simulink model "CITRIS_original"  (Simulink 7.4)
settings: Solver=FixedStepDiscrete  StartTime=0.0  StopTime=20  FixedStep=1  MaxStep=1  RelTol=1e-3
values from neighbouring files (symbols this model uses):
  mdot = [mdot controlInputHistory{i}(1,:)']    [CITRISBLOMSimulation.m]
  mdotmax = 740    [CITRISBLOMSimulation.m]
  mdotmin = 220    [CITRISBLOMSimulation.m]
  model =     [model.mat]
  vlv = [vlv controlInputHistory{i}(2,:)']    [CITRISBLOMSimulation.m]
undefined symbols (not defined in the file or in its folder): i, mdotTk, mdotvlv, mdotvlvk, Tk, TmaxSlack, TmaxV, TminSlack, TminV, wk, wk_1, wk_2
libraries: MPCMdlLib x19
settings Model: Creator=vichik  LastModifiedBy=Kyle
settings OptimizationCC: InitFltsAndDblsToZero=on

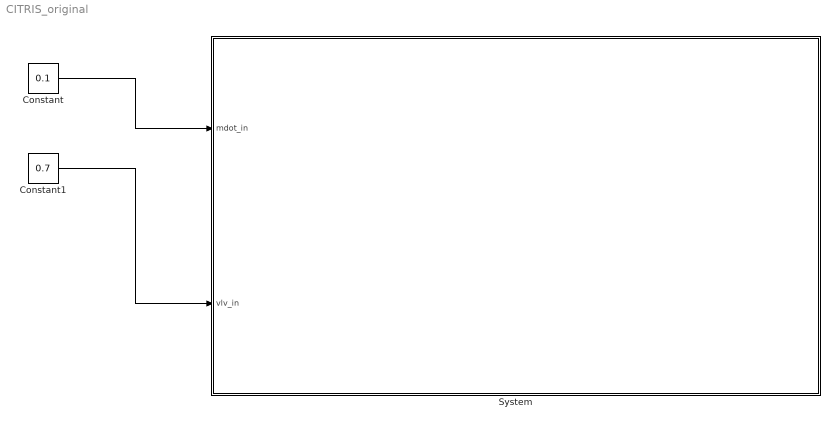
== system CITRIS_original ==
  Constant : Constant  Value=0.1
  Constant1 : Constant  Value=0.7
  System : Subsystem
  wires:
  Constant/1 -> System/1(mdot_in)
  Constant1/1 -> System/2(vlv_in)

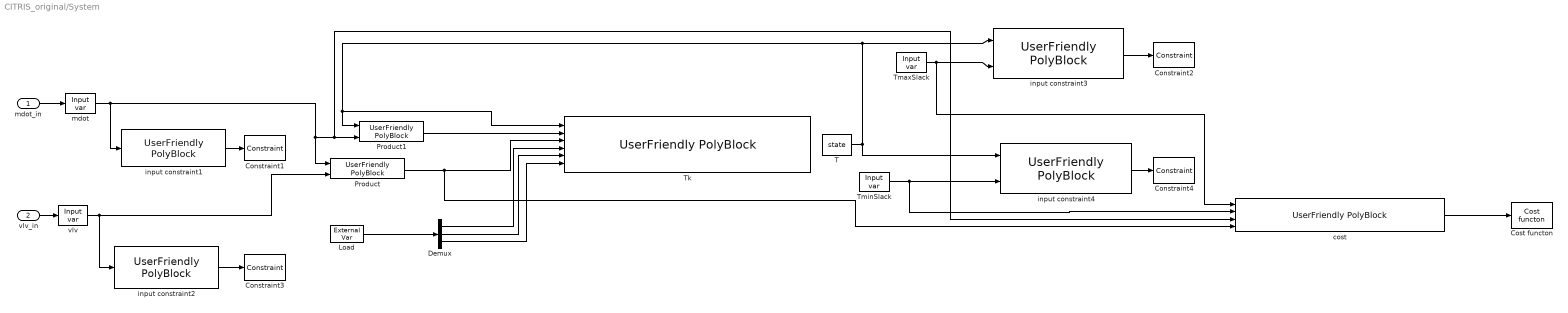
== system CITRIS_original/System ==
  mdot_in : Inport
  vlv_in : Inport  Port=2
  Constraint{1..4} (4 alike) : MPCMdlLib/Constraint  Tag=InequalBlock  CompareSign=< 0
  Cost functon : MPCMdlLib/Cost functon  Tag=OptCost
  Demux : Demux  Outputs=3
  Load : MPCMdlLib/External Var  Tag=OptExternal  SystemSampleTime=-1  step_ratio=1  save_name=BL_System_Load
  Product : MPCMdlLib/UserFriendly PolyBlock  Tag=PolyBlock  A="[1  1  ]"  C=[1 ]  gA=[0 0]  gC=1  input_type=Scalar  output_type=Scalar  port_names=mdot,vlv
  Product1 : MPCMdlLib/UserFriendly PolyBlock  Tag=PolyBlock  A="[1  1  ]"  C=[1 ]  gA=[0 0]  gC=1  input_type=Scalar  output_type=Scalar  port_names=Tk,mdot
  T : MPCMdlLib/state  Tag=OptState  SystemSampleTime=-1  init_val=T0  save_name=BL_System_T
  Tk : MPCMdlLib/UserFriendly PolyBlock  Tag=PolyBlock  A=[1 0 0 0 0 0;0 1 0 0 0 0;0 0 1 0 0 0;0 0 0 1 0 0;0 0 0 0 1 0;0 0 0 0 0 1;0 0 0 0 0 0]  C=[model{i}.A model{i}.B2 model{i}.B1 model{i}.W(1) model{i}.W(2) model{i}.W(3) model{i}.C]  gA=[0 0 0 0 0 0]  gC=1  input_type=Scalar  output_type=Scalar  port_names=Tk,mdotTk,mdotvlvk,wk,wk_1,wk_2
  TmaxSlack : MPCMdlLib/Input var  Tag=OptInput  SystemSampleTime=-1  step_ratio=1  save_name=BL_System_TmaxSlack
  TminSlack : MPCMdlLib/Input var  Tag=OptInput  SystemSampleTime=-1  step_ratio=1  save_name=BL_System_TminSlack
  "cost " : MPCMdlLib/UserFriendly PolyBlock  Tag=PolyBlock  A=[1 0 0 0;0 1 0 0;0 0 2 0;0 0 0 1]  C=[1 1 0.7*1e-6 1e-5]  gA=[0 0 0 0]  gC=1  input_type=Scalar  output_type=Scalar  port_names=TmaxV,TminV,mdot,mdotvlv
  input constraint1 : MPCMdlLib/UserFriendly PolyBlock  Tag=PolyBlock  A="[1  ;  0 ]"  C=[1 -mdotmax; -1 mdotmin]  gA="[0  ]"  gC=1  input_type=Scalar  output_type=Vector  port_names=mdot
  input constraint2 : MPCMdlLib/UserFriendly PolyBlock  Tag=PolyBlock  A=[1;0]  C="[1 -100; -1  0]"  gA=[0]  gC=1  input_type=Scalar  output_type=Vector  port_names=vlv
  input constraint3 : MPCMdlLib/UserFriendly PolyBlock  Tag=PolyBlock  A=[1 0;0 1;0 0]  C=[1 -1 -22;0 -1 0]  gA=[0 0]  gC=1  input_type=Scalar  output_type=Vector  port_names=Tk,TmaxSlack
  input constraint4 : MPCMdlLib/UserFriendly PolyBlock  Tag=PolyBlock  A=[1 0;0 1;0 0]  C=[-1 -1 20;0 -1 0]  gA=[0 0]  gC=1  input_type=Scalar  output_type=Vector  port_names=Tk,TminSlack
  mdot : MPCMdlLib/Input var  Tag=OptInput  SystemSampleTime=-1  step_ratio=1  save_name=BL_System_mdot
  vlv : MPCMdlLib/Input var  Tag=OptInput  SystemSampleTime=-1  step_ratio=1  save_name=BL_System_vlv
  wires:
  T/1 -> input constraint3/1, Product1/1, Tk/1, input constraint4/1
  mdot/1 -> "cost "/3, Product1/2, Product/1, input constraint1/1
  "cost "/1 -> Cost functon/1
  mdot_in/1 -> mdot/1
  input constraint1/1 -> Constraint1/1
  vlv_in/1 -> vlv/1
  vlv/1 -> Product/2, input constraint2/1
  input constraint2/1 -> Constraint3/1
  Load/1 -> Demux/1
  Demux/1 -> Tk/4
  Demux/2 -> Tk/5
  Demux/3 -> Tk/6
  Product1/1 -> Tk/2
  Product/1 -> "cost "/4, Tk/3
  input constraint3/1 -> Constraint2/1
  TmaxSlack/1 -> "cost "/1, input constraint3/2
  input constraint4/1 -> Constraint4/1
  TminSlack/1 -> "cost "/2, input constraint4/2
  ? -> T/1
